simulink model "Interactive Simulink"  (R2025a)
settings: Solver=VariableStepAuto  StartTime=0.0  StopTime=.1  FixedStep=5e-6  MaxStep=1e-6  RelTol=1e-3
libraries: spsBreakerLib x10, spsSeriesRLCBranchLib x8, spsRMSLib x4, spsACVoltageSourceLib x1, spsCurrentMeasurementLib x1, spsVoltageMeasurementLib x1, sps_lib x1
settings Model: Creator=KRISHNA  LastModifiedBy=KRISHNA

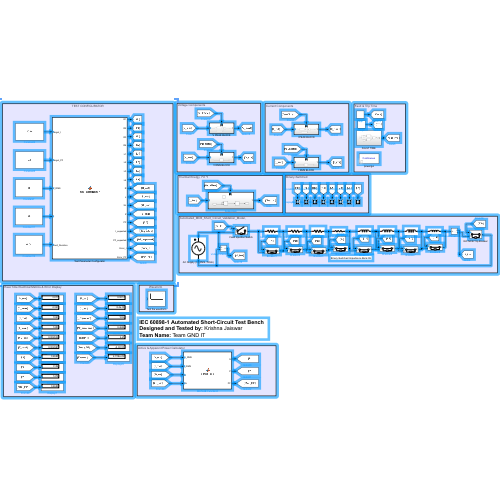
[thumbnail: Simulink's stored preview of the top-level diagram]
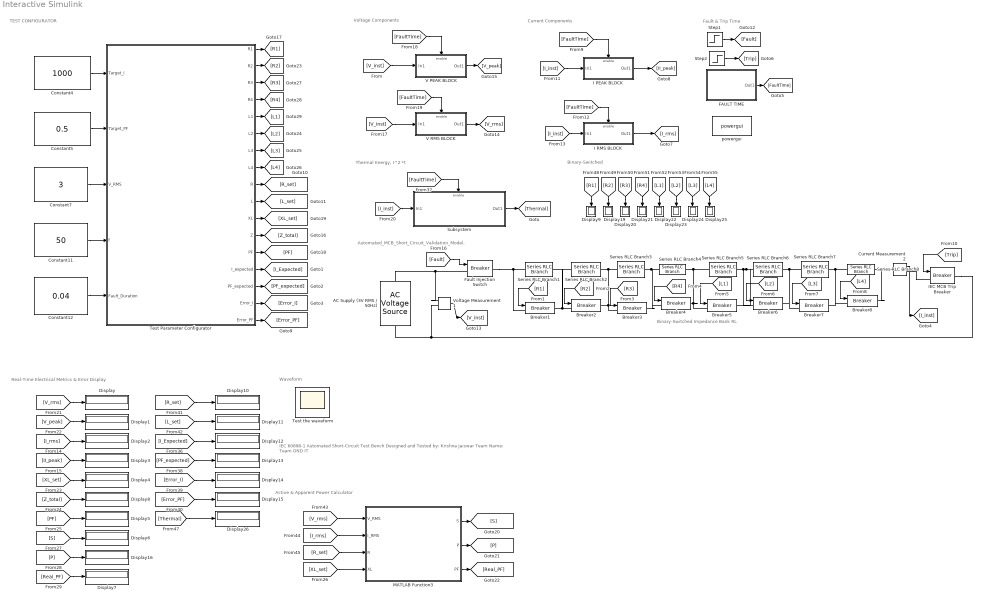
== system Interactive Simulink ==
  note: IEC 60898-1 Automated Short-Circuit Test Bench
      | Designed and Tested by: Krishna Jaiswar
      | Team Name: Team GND IT
  note: Automated_MCB_Short_Circuit_Validation_Model,
  note: Active & Apparent Power Calculator
  note: Waveform
  note: Real-Time Electrical Metrics & Error Display
  note: TEST CONFIGURATOR
  note: Binary-Switched
  note: Thermal Energy, I^2 *t
  note: Fault & Trip Time
  note: Voltage Components
  note: Binary-Switched Impedance Bank RL
  note: Current Components
  AC Supply (3V RMS / 50Hz) : spsACVoltageSourceLib/AC Voltage Source  Amplitude=4.3426  Phase=0  Frequency=50  SampleTime=0  Measurements=None  BusType=swing  Pref=10e3  Qref=0  Qmin=-inf  Qmax=+inf
  Breaker1 : spsBreakerLib/Breaker  InitialState=1  SwitchingTimes="[1/60  5/60]"  External=on  BreakerResistance=1e-6  SnubberResistance=1e6  SnubberCapacitance=inf  Measurements=None  MoreParameters=on  NoBreakLoop=off
  Breaker{2..8} (7 alike) : spsBreakerLib/Breaker  InitialState=1  SwitchingTimes="[1/60  5/60]"  External=on  BreakerResistance=2e-6  SnubberResistance=1e6  SnubberCapacitance=inf  Measurements=None  MoreParameters=on  NoBreakLoop=off
  Constant11 : Constant  Value=50
  Constant12 : Constant  Value=0.04
  Constant4 : Constant  Value=1000
  Constant5 : Constant  Value=0.5
  Constant7 : Constant  Value=3
  Current Measurement2 : spsCurrentMeasurementLib/Current Measurement  PhasorSimulation=off  OutputType=Complex  PSBequivalent=0
  Display{,1..16,19..26} (25 alike) : Display
  FAULT TIME : Subsystem
  Fault Injection Switch : spsBreakerLib/Breaker  InitialState=0  SwitchingTimes="[1/60  5/60]"  External=on  BreakerResistance=1e-6  SnubberResistance=1e6  SnubberCapacitance=inf  Measurements=None  MoreParameters=on  NoBreakLoop=off
  I PEAK BLOCK : Subsystem  TreatAsAtomicUnit=on
  I RMS BLOCK : Subsystem  TreatAsAtomicUnit=on
  IEC MCB Trip Breaker : spsBreakerLib/Breaker  InitialState=1  SwitchingTimes="[1/60  5/60]"  External=on  BreakerResistance=1e-6  SnubberResistance=1e6  SnubberCapacitance=inf  Measurements=None  MoreParameters=on  NoBreakLoop=off
  MATLAB Function3 : MATLAB Function  TreatAsAtomicUnit=on
  Series RLC Branch1 : spsSeriesRLCBranchLib/Series RLC Branch  LConnTagsString=__new0  RConnTagsString=__new0  BranchType=R  Resistance=0.2e-3  Inductance=7.8e-6  SetiL0=off  InitialCurrent=0  Capacitance=1e-6  Setx0=off  InitialVoltage=0  Measurements=None
  Series RLC Branch2 : spsSeriesRLCBranchLib/Series RLC Branch  LConnTagsString=__new0  RConnTagsString=__new0  BranchType=R  Resistance=0.4e-3  Inductance=7.8e-6  SetiL0=off  InitialCurrent=0  Capacitance=1e-6  Setx0=off  InitialVoltage=0  Measurements=None
  Series RLC Branch3 : spsSeriesRLCBranchLib/Series RLC Branch  LConnTagsString=__new0  RConnTagsString=__new0  BranchType=R  Resistance=0.8e-3  Inductance=7.8e-6  SetiL0=off  InitialCurrent=0  Capacitance=1e-6  Setx0=off  InitialVoltage=0  Measurements=None
  Series RLC Branch4 : spsSeriesRLCBranchLib/Series RLC Branch  LConnTagsString=__new0  RConnTagsString=__new0  BranchType=R  Resistance=1.6e-3  Inductance=7.8e-6  SetiL0=off  InitialCurrent=0  Capacitance=1e-6  Setx0=off  InitialVoltage=0  Measurements=None
  Series RLC Branch5 : spsSeriesRLCBranchLib/Series RLC Branch  LConnTagsString=__new0  RConnTagsString=__new0  BranchType=L  Resistance=0.2e-3  Inductance=0.6e-6  SetiL0=off  InitialCurrent=0  Capacitance=1e-6  Setx0=off  InitialVoltage=0  Measurements=None
  Series RLC Branch6 : spsSeriesRLCBranchLib/Series RLC Branch  LConnTagsString=__new0  RConnTagsString=__new0  BranchType=L  Resistance=0.4e-3  Inductance=1.2e-6  SetiL0=off  InitialCurrent=0  Capacitance=1e-6  Setx0=off  InitialVoltage=0  Measurements=None
  Series RLC Branch7 : spsSeriesRLCBranchLib/Series RLC Branch  LConnTagsString=__new0  RConnTagsString=__new0  BranchType=L  Resistance=0.8e-3  Inductance=2.4e-6  SetiL0=off  InitialCurrent=0  Capacitance=1e-6  Setx0=off  InitialVoltage=0  Measurements=None
  Series RLC Branch8 : spsSeriesRLCBranchLib/Series RLC Branch  LConnTagsString=__new0  RConnTagsString=__new0  BranchType=L  Resistance=1.6e-3  Inductance=4.8e-6  SetiL0=off  InitialCurrent=0  Capacitance=1e-6  Setx0=off  InitialVoltage=0  Measurements=None
  Step1 : Step  Time=0.02  SampleTime=0  ZeroCross=off
  Step2 : Step  Time=0.06  Before=1  After=0  SampleTime=0  ZeroCross=off
  Subsystem : Subsystem
  Test Parameter Configurator : MATLAB Function  TreatAsAtomicUnit=on
  Test the waveform : Scope
  V PEAK BLOCK : Subsystem  TreatAsAtomicUnit=on
  V RMS BLOCK : Subsystem  TreatAsAtomicUnit=on
  Voltage Measurement1 : spsVoltageMeasurementLib/Voltage Measurement  PhasorSimulation=off  OutputType=Complex  PSBequivalent=0
  powergui : sps_lib/powergui  Priority=1  SimulationMode=Continuous  SampleTime=5e-6  frequency=60  Iterations=50  frequencyindice=50  Pbase=100e6  ErrMax=1e-4  UnitsV=kV  UnitsW=MW  buscounter=0  FunctionMessages=off  echomessages=off  EnableUseOfTLC=off  CurrentSourceSwitches=off  DisableSnubberDevices=off  DisableRonSwitches=off  DisableVfSwitches=off  DisplayEquations=off  AutomaticDiscreteSolvers=off  SolverType=Tustin/Backward Euler (TBE)  Interpol=off  ExternalGateDelay=off  methode=off  Ts=100  x0status=blocks  SPID=on  SwTol=0  HookPort=off  NonlinearTolerance=1e-4  nMaxIteration=100  ContinueOnMaxIteration=off  RestoreLinks=warning  ResistiveCurrentMeasurement=off  Frange=[0:2:500]  Ylog=off  Xlog=on  ShowGrid=off  save=off  variable=ZData  structure=0  ZoomFFT=off  StartTime=0.0  cycles=1  DisplayStyle=1  fundamental=60  FreqAxis=off  MaxFrequency=1000  frequencyindicesteady=1  RmsSteady=1  display=off
  wires:
  [L1] -> Breaker5/1
  [L2] -> Breaker6/1
  [L3] -> Breaker7/1
  [L4] -> Breaker8/1
  [R4] -> Breaker4/1
  [R3] -> Breaker3/1
  [R2] -> Breaker2/1
  [R1] -> Breaker1/1
  FAULT TIME/1(Out1) -> [FaultTime]
  [FaultTime] -> I PEAK BLOCK/Enable
  [I_inst] -> I PEAK BLOCK/1(In1)
  [FaultTime] -> I RMS BLOCK/Enable
  [I_inst] -> I RMS BLOCK/1(In1)
  Current Measurement2/1 -> [I_inst]
  Step2/1 -> [Trip]
  [Trip] -> IEC MCB Trip Breaker/1
  Step1/1 -> [Fault]
  [Fault] -> Fault Injection Switch/1
  Voltage Measurement1/1 -> [V_inst]
  [V_inst] -> V PEAK BLOCK/1(In1)
  [FaultTime] -> V PEAK BLOCK/Enable
  [V_inst] -> V RMS BLOCK/1(In1)
  [FaultTime] -> V RMS BLOCK/Enable
  [V_rms] -> Display/1
  [V_peak] -> Display1/1
  [I_rms] -> Display2/1
  [II_peak] -> Display3/1
  V PEAK BLOCK/1(Out1) -> [V_peak]
  V RMS BLOCK/1(Out1) -> [V_rms]
  [XL_set] -> Display4/1
  [I_inst] -> Subsystem/1(In1)
  [FaultTime] -> Subsystem/Enable
  Subsystem/1(Out1) -> [Thermal]
  I RMS BLOCK/1(Out1) -> [I_rms]
  I PEAK BLOCK/1(Out1) -> [II_peak]
  Test Parameter Configurator/1(R1) -> [R1]
  Test Parameter Configurator/2(R2) -> [R2]
  Test Parameter Configurator/3(R3) -> [R3]
  Test Parameter Configurator/4(R4) -> [R4]
  Test Parameter Configurator/5(L1) -> [L1]
  Test Parameter Configurator/6(L2) -> [L2]
  Test Parameter Configurator/7(L3) -> [L3]
  Test Parameter Configurator/8(L4) -> [L4]
  Constant4/1 -> Test Parameter Configurator/1(Target_I)
  Constant5/1 -> Test Parameter Configurator/2(Target_PF)
  Constant7/1 -> Test Parameter Configurator/3(V_RMS)
  Constant11/1 -> Test Parameter Configurator/4(f)
  Constant12/1 -> Test Parameter Configurator/5(Fault_Duration)
  [R_set] -> Display10/1
  [L_set] -> Display11/1
  [I_Expected] -> Display12/1
  [PF_expected] -> Display13/1
  [Error_I] -> Display14/1
  [Error_PF] -> Display15/1
  Test Parameter Configurator/9(R) -> [R_set]
  Test Parameter Configurator/10(L) -> [L_set]
  Test Parameter Configurator/14(I_expected) -> [I_Expected]
  Test Parameter Configurator/15(PF_expected) -> [PF_expected]
  Test Parameter Configurator/16(Error_I) -> [Error_I]
  Test Parameter Configurator/17(Error_PF) -> [Error_PF]
  [V_rms] -> MATLAB Function3/1(V_RMS)
  [I_rms] -> MATLAB Function3/2(I_RMS)
  [R_set] -> MATLAB Function3/3(R)
  [R1] -> Display9/1
  [R2] -> Display19/1
  [R3] -> Display20/1
  [R4] -> Display21/1
  [L1] -> Display22/1
  [L2] -> Display23/1
  [L3] -> Display24/1
  [L4] -> Display25/1
  [Thermal] -> Display26/1
  Test Parameter Configurator/11(XL) -> [XL_set]
  Test Parameter Configurator/13(PF) -> [PF]
  Test Parameter Configurator/12(Z) -> [Z_total]
  [Z_total] -> Display8/1
  [XL_set] -> MATLAB Function3/4(XL)
  MATLAB Function3/1(S) -> [S]
  MATLAB Function3/2(P) -> [P]
  MATLAB Function3/3(PF) -> [Real_PF]
  [S] -> Display6/1
  [P] -> Display16/1
  [Real_PF] -> Display7/1
  [PF] -> Display5/1
  connections:
  Current Measurement2/LConn1 -- Breaker8/RConn1 -- Series RLC Branch8/RConn1
  IEC MCB Trip Breaker/RConn1 -- AC Supply (3V RMS / 50Hz)/LConn1 -- Voltage Measurement1/LConn2
  Series RLC Branch7/LConn1 -- Breaker7/LConn1 -- Breaker6/RConn1 -- Series RLC Branch6/RConn1
  Series RLC Branch8/LConn1 -- Breaker8/LConn1 -- Breaker7/RConn1 -- Series RLC Branch7/RConn1
  Series RLC Branch6/LConn1 -- Series RLC Branch5/RConn1 -- Breaker6/LConn1 -- Breaker5/RConn1
  Current Measurement2/RConn1 -- IEC MCB Trip Breaker/LConn1
  Voltage Measurement1/LConn1 -- AC Supply (3V RMS / 50Hz)/RConn1 -- Fault Injection Switch/LConn1
  Series RLC Branch3/RConn1 -- Series RLC Branch4/LConn1 -- Breaker3/RConn1 -- Breaker4/LConn1
  Breaker2/RConn1 -- Breaker3/LConn1 -- Series RLC Branch3/LConn1 -- Series RLC Branch2/RConn1
  Breaker1/RConn1 -- Series RLC Branch2/LConn1 -- Series RLC Branch1/RConn1 -- Breaker2/LConn1
  Breaker4/RConn1 -- Series RLC Branch5/LConn1 -- Series RLC Branch4/RConn1 -- Breaker5/LConn1
  Series RLC Branch1/LConn1 -- Breaker1/LConn1 -- Fault Injection Switch/RConn1

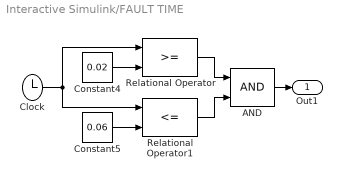
== system Interactive Simulink/FAULT TIME ==
  AND : Logic  IconShape=distinctive  AllPortsSameDT=off  OutDataTypeStr=boolean
  Clock : Clock
  Constant4 : Constant  Value=0.02
  Constant5 : Constant  Value=0.06
  Relational Operator : RelationalOperator  OutDataTypeStr=boolean  RndMeth=Simplest  InputSameDT=off
  Relational Operator1 : RelationalOperator  Operator=<=  OutDataTypeStr=boolean  RndMeth=Simplest  InputSameDT=off
  Out1 : Outport
  wires:
  Clock/1 -> Relational Operator1/1, Relational Operator/1
  Relational Operator1/1 -> AND/2
  Constant5/1 -> Relational Operator1/2
  Relational Operator/1 -> AND/1
  AND/1 -> Out1/1
  Constant4/1 -> Relational Operator/2

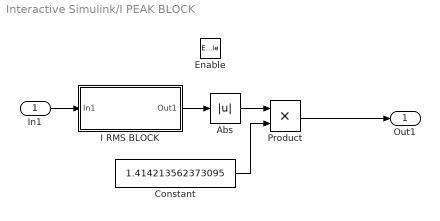
== system Interactive Simulink/I PEAK BLOCK ==
  In1 : Inport
  Enable : EnablePort
  Abs : Abs  SaturateOnIntegerOverflow=off
  Constant : Constant  Value=1.414213562373095
  I RMS BLOCK : Subsystem  TreatAsAtomicUnit=on
  Product : Product
  Out1 : Outport
  wires:
  Constant/1 -> Product/2
  Product/1 -> Out1/1
  I RMS BLOCK/1(Out1) -> Abs/1
  In1/1 -> I RMS BLOCK/1(In1)
  Abs/1 -> Product/1

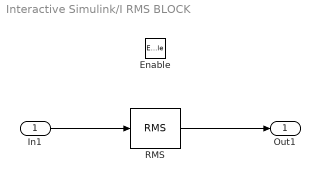
== system Interactive Simulink/I RMS BLOCK ==
  In1 : Inport
  Enable : EnablePort
  RMS : spsRMSLib/RMS  TrueRMS=on  Freq=50  RMSInit=0  Ts=0
  Out1 : Outport
  wires:
  RMS/1 -> Out1/1
  In1/1 -> RMS/1

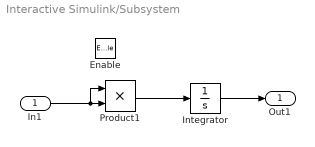
== system Interactive Simulink/Subsystem ==
  In1 : Inport
  Enable : EnablePort
  Integrator : Integrator
  Product1 : Product
  Out1 : Outport
  wires:
  Product1/1 -> Integrator/1
  Integrator/1 -> Out1/1
  In1/1 -> Product1/1, Product1/2

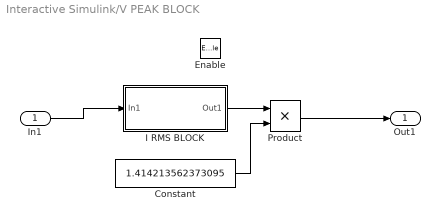
== system Interactive Simulink/V PEAK BLOCK ==
  In1 : Inport
  Enable : EnablePort
  Constant : Constant  Value=1.414213562373095
  I RMS BLOCK : Subsystem  TreatAsAtomicUnit=on
  Product : Product
  Out1 : Outport
  wires:
  In1/1 -> I RMS BLOCK/1(In1)
  I RMS BLOCK/1(Out1) -> Product/1
  Product/1 -> Out1/1
  Constant/1 -> Product/2

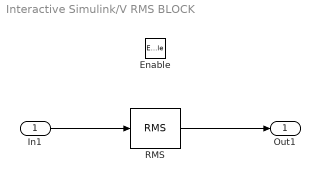
== system Interactive Simulink/V RMS BLOCK ==
  In1 : Inport
  Enable : EnablePort
  RMS : spsRMSLib/RMS  TrueRMS=on  Freq=50  RMSInit=120  Ts=0
  Out1 : Outport
  wires:
  In1/1 -> RMS/1
  RMS/1 -> Out1/1

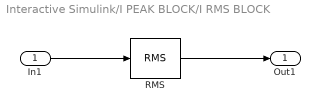
== system Interactive Simulink/I PEAK BLOCK/I RMS BLOCK ==
  In1 : Inport
  RMS : spsRMSLib/RMS  TrueRMS=on  Freq=50  RMSInit=0  Ts=0
  Out1 : Outport
  wires:
  In1/1 -> RMS/1
  RMS/1 -> Out1/1

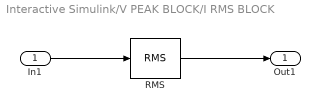
== system Interactive Simulink/V PEAK BLOCK/I RMS BLOCK ==
  In1 : Inport
  RMS : spsRMSLib/RMS  TrueRMS=on  Freq=50  RMSInit=120  Ts=0
  Out1 : Outport
  wires:
  RMS/1 -> Out1/1
  In1/1 -> RMS/1

== matlab function Interactive Simulink/Test Parameter Configurator ==
  data: Target_I input; R1 output; Target_PF input; V_RMS input; f input; Fault_Duration input; R2 output; R3 output; R4 output; L1 output; L2 output; L3 output; L4 output; R output; L output; XL output; Z output; PF output; I_expected output; PF_expected output; Error_I output; Error_PF output
function [R1, R2, R3, R4, L1, L2, L3, L4, ...
          R, L, XL, Z, PF, ...
          I_expected, PF_expected, Error_I, Error_PF] = ...
          test_configurator(Target_I, Target_PF, V_RMS, f, Fault_Duration)
% =========================================================
% COMBINED TEST CONFIGURATION & IMPEDANCE CALCULATOR
% 1 = bypass ON  -> component removed
% 0 = bypass OFF -> component included
% =========================================================

%% Component values
R_values = [0.2 0.4 0.8 1.6]*1e-3;
L_values = [0.6 1.2 2.4 4.8]*1e-6;

%% INITIALIZE ALL OUTPUT VARIABLES
best_error = inf;
R_bits = zeros(1,4);
L_bits = zeros(1,4);
R_set = 0;
L_set = 0;
I_expected = 0;
PF_expected = 0;

%% SEARCH ALL 256 COMBINATIONS
for r = 0:15
    % Resistor switch states
    rb = [bitget(r,1), bitget(r,2), ...
          bitget(r,3), bitget(r,4)];
    R_curr = sum((1 - rb) .* R_values);
    
    for l = 0:15
        % Inductor switch states
        lb = [bitget(l,1), bitget(l,2), ...
              bitget(l,3), bitget(l,4)];
        L_curr = sum((1 - lb) .* L_values);
        
        % Inductive reactance & Impedance
        XL_curr = 2 * pi * f * L_curr;
        Z_curr = sqrt(R_curr^2 + XL_curr^2);
        
        if Z_curr > 0
            I_curr = V_RMS / Z_curr;
            PF_curr = R_curr / Z_curr;
            
            % Error calculations
            current_error = abs(I_curr - Target_I) / Target_I;
            pf_error = abs(PF_curr - Target_PF);
            total_error = current_error + pf_error;
            
            % Store best combination
            if total_error < best_error
                best_error = total_error;
                R_set = R_curr;
                L_set = L_curr;
                R_bits = rb;
                L_bits = lb;
                I_expected = I_curr;
                PF_expected = PF_curr;
            end
        end
    end
end

%% OUTPUT SWITCH STATES
R1 = R_bits(1);
R2 = R_bits(2);
R3 = R_bits(3);
R4 = R_bits(4);
L1 = L_bits(1);
L2 = L_bits(2);
L3 = L_bits(3);
L4 = L_bits(4);

%% CALCULATE FINAL IMPEDANCE & POWER FACTOR METRICS
R = R_set;
L = L_set;
XL = 2 * pi * f * L;
Z = sqrt(R^2 + XL^2);

if Z > 0
    PF = R / Z;
else
    PF = 0;
end

%% FINAL ERRORS
Error_I = I_expected - Target_I;
Error_PF = PF_expected - Target_PF;

end

== matlab function Interactive Simulink/MATLAB Function3 ==
  data: V_RMS input; S output; P output; I_RMS input; R input; XL input; PF output
function [S,P,PF] = power_calc(V_RMS,I_RMS,R,XL)

% Apparent power
S = V_RMS * I_RMS;

% Total impedance
Z = sqrt(R^2 + XL^2);

% True power
if Z > 0
    PF = R / Z;
else
    PF = 0;
end

% Active power
P = S * PF;

end
